simulink model "estimator1"  (Simulink 8.1)
settings: Solver=ode45  StartTime=0.0  StopTime=10.0  RelTol=1e-3
undefined symbols (not defined in the file or in its folder): A, C, L, x1, x1h
libraries: Is_equal_scalar x1, goal x1
settings Model: Creator=dejanira  LastModifiedBy=dejanira
settings DataIOCC: SignalLoggingSaveFormat=Dataset
settings OptimizationCC: ExpressionDepthLimit=128
settings DebuggingCC: FcnCallInpInsideContextMsg=EnableAllAsError
settings GRTTargetCC: CombineOutputUpdateFcns=on  GRTInterface=off

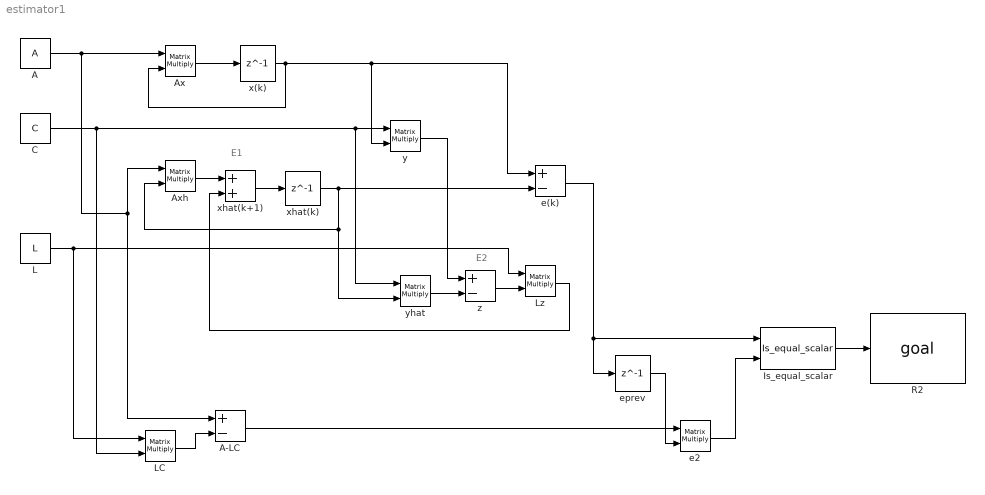
== system estimator1 ==
  note: E1
  note: E2
  A : Constant  Value=A  VectorParams1D=off
  A-LC : Sum  Inputs=+-
  Ax : Product  Multiplication=Matrix(*)
  Axh : Product  Multiplication=Matrix(*)
  C : Constant  Value=C  VectorParams1D=off
  Is_equal_scalar : Is_equal_scalar/Is_equal_scalar  SystemSampleTime=-1
  L : Constant  Value=L  VectorParams1D=off
  LC : Product  Multiplication=Matrix(*)
  Lz : Product  Multiplication=Matrix(*)
  R2 : goal/goal  SystemSampleTime=-1
  e(k) : Sum  Inputs=+-
  e2 : Product  Multiplication=Matrix(*)
  eprev : Delay  DelayLength=1  InitialCondition=x1  SampleTime=0.1
  x(k) : Delay  DelayLength=1  InitialCondition=x1  SampleTime=0.1
  xhat(k) : Delay  DelayLength=1  InitialCondition=x1h
  xhat(k+1) : Sum
  y : Product  Multiplication=Matrix(*)
  yhat : Product  Multiplication=Matrix(*)
  z : Sum  Inputs=+-
  wires:
  A/1 -> A-LC/1, Axh/1, Ax/1
  Ax/1 -> x(k)/1
  xhat(k)/1 -> e(k)/2, yhat/2, Axh/2
  xhat(k+1)/1 -> xhat(k)/1
  z/1 -> Lz/2
  x(k)/1 -> Ax/2, y/2, e(k)/1
  L/1 -> LC/1, Lz/1
  Is_equal_scalar/1 -> R2/1
  Axh/1 -> xhat(k+1)/1
  Lz/1 -> xhat(k+1)/2
  eprev/1 -> e2/2
  e2/1 -> Is_equal_scalar/2
  e(k)/1 -> Is_equal_scalar/1, eprev/1
  A-LC/1 -> e2/1
  C/1 -> LC/2, y/1, yhat/1
  y/1 -> z/1
  yhat/1 -> z/2
  LC/1 -> A-LC/2
